simulink model "Vorlage_backcalc"  (R2024a)
settings: Solver=ode45  StartTime=0.0  StopTime=20  FixedStep=1e-2  RelTol=1e-4  AbsTol=1e-4
values from neighbouring files (symbols this model uses):
  ka = 1    [matlab_verification.m]
  Kp = 10    [matlab_verification.m]
  Td = 0.2972    [matlab_verification.m]
  Ti = 9.5608    [matlab_verification.m]
libraries: cstblocks x1
settings Model: Creator=bhir  LastModifiedBy=Flo
settings SolverCC: AlgebraicLoopSolver=TrustRegion
settings DataIOCC: ReturnWorkspaceOutputs=off
settings DebuggingCC: UnconnectedInputMsg=warning  UnconnectedOutputMsg=warning  UnconnectedLineMsg=warning  ArithmeticOperatorsInVariantConditions=warning
settings SFSimCC: SimUseLocalCustomCode=off  CustomCodeUndefinedFunction=UseInterfaceOnly
settings RTWCC: RTWUseLocalCustomCode=off  GPUComputeCapability=3.5  DLArmComputeVersion=19.05
settings CodeAppCC: StateflowObjectComments=on

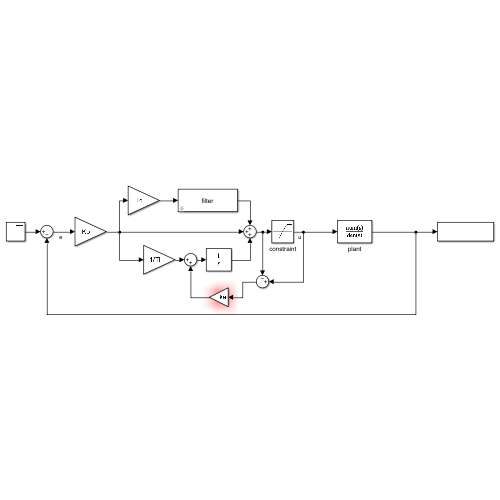
[thumbnail: Simulink's stored preview of the top-level diagram]
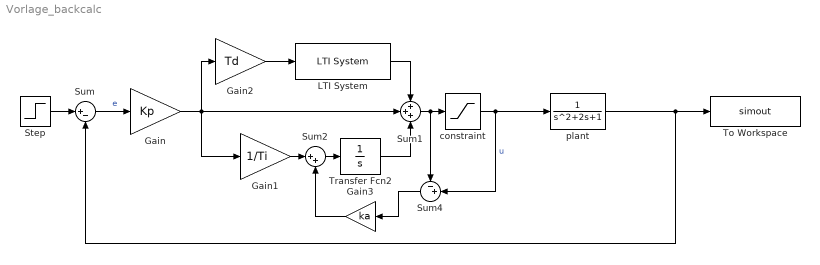
== system Vorlage_backcalc ==
  Gain : Gain  Gain=Kp
  Gain1 : Gain  Gain=1/Ti
  Gain2 : Gain  Gain=Td
  Gain3 : Gain  Gain=ka
  LTI System : cstblocks/LTI System  sys=filter  IC=[]  PadeOrder=0
  Step : Step  Time=0  SampleTime=0
  Sum : Sum  Inputs=|+-
  Sum1 : Sum  Inputs=+++
  Sum2 : Sum  Inputs=|++
  Sum4 : Sum  Inputs=-+|
  To Workspace : ToWorkspace  VariableName=simout  SaveFormat=Structure With Time  SampleTime=-1
  Transfer Fcn2 : TransferFcn  Denominator=[1 0]
  constraint : Saturate  UpperLimit=2  LowerLimit=-2
  plant : TransferFcn
  wires:
  Step/1 -> Sum/1
  Sum/1 -> Gain/1  "e"
  LTI System/1 -> Sum1/1
  Gain2/1 -> LTI System/1
  Sum1/1 -> Sum4/1, constraint/1
  Transfer Fcn2/1 -> Sum1/3
  constraint/1 -> plant/1, Sum4/2  "u"
  plant/1 -> To Workspace/1, Sum/2
  Gain/1 -> Gain2/1, Gain1/1, Sum1/2
  Gain1/1 -> Sum2/1
  Sum2/1 -> Transfer Fcn2/1
  Sum4/1 -> Gain3/1
  Gain3/1 -> Sum2/2
